simulink model "voltages_of_parallel_RCs"  (Simulink 8.9)
settings: Solver=ode45  StartTime=0.0  StopTime=10.0  RelTol=1e-3  EnableMultiTasking=on
settings Model: SuppressorTable=22 serialization::archive 11 0 6 0 0 0 0 0  Creator=hlopez5  LastModifiedBy=judithlopez
settings DataIOCC: SignalLoggingSaveFormat=Dataset
settings DebuggingCC: UnderspecifiedInitializationDetection=Simplified  MergeDetectMultiDrivingBlocksExec=error  SolverPrmCheckMsg=warning  FcnCallInpInsideContextMsg=error
settings GRTTargetCC: CombineOutputUpdateFcns=on  GRTInterface=off

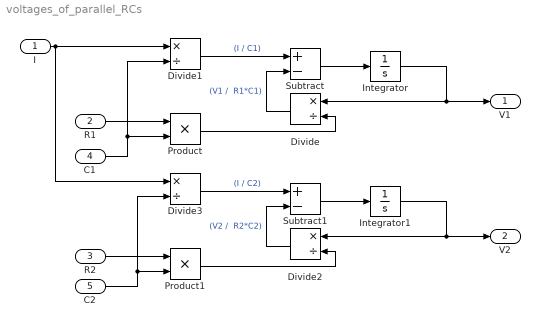
== system voltages_of_parallel_RCs ==
  I : Inport
  R1 : Inport  Port=2
  R2 : Inport  Port=3
  C1 : Inport  Port=4
  C2 : Inport  Port=5
  Divide{,1..3} (4 alike) : Product  Inputs=*/
  Integrator : Integrator
  Integrator1 : Integrator
  Product : Product
  Product1 : Product
  Subtract : Sum  Inputs=+-
  Subtract1 : Sum  Inputs=+-
  V1 : Outport
  V2 : Outport  Port=2
  wires:
  R1/1 -> Product/1
  C1/1 -> Product/2, Divide1/2
  Product/1 -> Divide/2
  Divide/1 -> Subtract/2  "(V1 /  R1*C1)"
  Subtract/1 -> Integrator/1
  Integrator/1 -> Divide/1, V1/1
  Divide1/1 -> Subtract/1  "(I / C1)"
  R2/1 -> Product1/1
  C2/1 -> Product1/2, Divide3/2
  Product1/1 -> Divide2/2
  Divide2/1 -> Subtract1/2  "(V2 /  R2*C2)"
  Subtract1/1 -> Integrator1/1
  Integrator1/1 -> V2/1, Divide2/1
  I/1 -> Divide3/1, Divide1/1
  Divide3/1 -> Subtract1/1  "(I / C2)"
